simulink model "EvPowertrainController2EM_r2_23a"  (R2023a)
settings: configuration reference "VehicleFixed10ms" (kept outside this file)
model workspace (MAT data in the model file):
  CtrlVcuAccelTrqScaleFctr = [0 0.5 0.8 1 1]
  CtrlVcuBattPnlty = 10000000
  CtrlVcuBattSOCBpts = [0 20 60 80 100]
  CtrlVcuCnstrntPnltyFctr = 10000000
  CtrlVcuEMPnlty = 100
  CtrlVcuEMTrqSplitGrid = 200
  CtrlVcuMaxAccelG = 1
  CtrlVcuMaxDecelG = -1.5
  CtrlVcuPwrDeltaPnlty = 10
  CtrlVcuRegenTrqScaleFctr = [1 0.8 0.5 0.3 0]
  CtrlVcuRoadMuEst = 0.8
  CtrlVcuSftyFctr = 0.9
  CtrlVcuTracPwrErrPnlty = 6
  CtrlVcuTrqVecBrkThresh = 0.01
  CtrlVcuTrqVecIGain = 0
  CtrlVcuTrqVecMinTrq = 25
  CtrlVcuTrqVecPGain = -2000
  CtrlVcuTrqVecSteerThresh = 0.349065850399
  CtrlVcuTrqVecVelThresh = 2.5
  N_P0 = 3
undefined symbols (not defined in the file): CtrlVcuEvChrgLmtBpt, CtrlVcuEvRegenBrkCutOff, CtrlVcuEvSocBpt, eff, EnvGrvty, PlntBrkActrBoreFrnt, PlntBrkFrntBias, PlntBrkKinFricCffFrnt, PlntBrkNumPadsFrnt, PlntBrkPadMeanRadiusFrnt, PlntBrkPrsFctr, PlntBrkRearBias, PlntDiffrntl2Eff, PlntDiffrntl2Ratio, PlntDiffrntlEff, PlntDiffrntlRatio, PlntEM1EffTbl, PlntEM1Spd, PlntEM1Trq, PlntEM1TrqEff, PlntEM2EffTbl, PlntEM2Spd, PlntEM2Trq, PlntEM2TrqEff, PlntEM3EffTbl, PlntEM3Spd, PlntEM3Trq, PlntEM3TrqEff, PlntEMWhlGearEffFL, PlntEMWhlGearEffRL, PlntEMWhlGearRatioFL, PlntEMWhlGearRatioRL, PlntTransEffSpdBpt, PlntTransEffTbl, PlntTransEffTempBpt, PlntTransEffTrqBpt, PlntTransGearNumVect, PlntTransGearRatioVect, PlntVehCGHgtAxl, PlntVehDstCGFrntAxl, PlntVehDstCGRearAxl, PlntVehMass, PlntWhlLdRadius, RegenEnd, RegenStrt
libraries: simulink x28, autolibutils x4, slpidlib x2
(part 5 of 6)

== system EvPowertrainController2EM_r2_23a/Energy Management/Calculate Average EMSpd and Wheel Torque Curves for Front and Rear Axles/2EM/EMTrq2WhlTrqRear/Transmission/Diff Eta ==
  SpdIn : Inport
  TrqIn : Inport  Port=2
  Constant : Constant  Value=PlntDiffrntl2Eff
  Constant1 : Constant  SampleTime=-1
  Constant2 : Constant  Value=-1  SampleTime=-1
  Math Function1 : Math  Operator=pow  SignedPower=on  OutputSignalType=real
  Product1 : Product
  Switch2 : Switch  SaturateOnIntegerOverflow=off  InputSameDT=off
  eta : Outport  VectorParamsAs1DForOutWhenUnconnected=off
  wires:
  TrqIn/1 -> Product1/1
  Math Function1/1 -> eta/1
  Switch2/1 -> Math Function1/2
  Product1/1 -> Switch2/2
  Constant1/1 -> Switch2/1
  Constant2/1 -> Switch2/3
  Constant/1 -> Math Function1/1
  SpdIn/1 -> Product1/2

== system EvPowertrainController2EM_r2_23a/Energy Management/Calculate Average EMSpd and Wheel Torque Curves for Front and Rear Axles/2EM/EMTrq2WhlTrqRear/Transmission/Trans Eta ==
  TrqIn : Inport
  SpdIn : Inport  Port=2
  Gear : Inport  Port=3
  Abs1 : Abs  SaturateOnIntegerOverflow=off
  Constant : Constant  Value=PlntTransEffTempBpt(1)
  Constant1 : Constant  SampleTime=-1
  Constant2 : Constant  Value=-1  SampleTime=-1
  Eta 4D : Lookup_n-D  NumberOfTableDimensions=4  LookupTableObject=''  BreakpointsForDimension1=PlntTransEffTrqBpt  BreakpointsForDimension2=PlntTransEffSpdBpt  BreakpointsForDimension3=PlntTransGearNumVect  BreakpointsForDimension4=PlntTransEffTempBpt  Table=PlntTransEffTbl  ExtrapMethod=Clip  InternalRulePriority=Speed  RndMeth=Simplest
      settings: InputPortMap=u0,u1,u2,u3
  Math Function1 : Math  Operator=pow  SignedPower=on  OutputSignalType=real
  Product1 : Product
  Switch2 : Switch  SaturateOnIntegerOverflow=off  InputSameDT=off
  eta : Outport  VectorParamsAs1DForOutWhenUnconnected=off
  wires:
  Constant/1 -> Eta 4D/4
  Gear/1 -> Eta 4D/3
  SpdIn/1 -> Eta 4D/2, Product1/2
  Eta 4D/1 -> Math Function1/1
  Constant2/1 -> Switch2/3
  Constant1/1 -> Switch2/1
  Product1/1 -> Switch2/2
  Switch2/1 -> Math Function1/2
  Abs1/1 -> Eta 4D/1
  Math Function1/1 -> eta/1
  TrqIn/1 -> Abs1/1, Product1/1

== system EvPowertrainController2EM_r2_23a/Energy Management/Calculate Average EMSpd and Wheel Torque Curves for Front and Rear Axles/3EM Dual Front/EMTrq2WhlTrqFrnt/No Transmission/Gear Eta ==
  note: Pwr >= 0, v = 1
      | Pwr < 0, v= -1
  SpdIn : Inport
  TrqIn : Inport  Port=2
  Constant : Constant  Value=PlntEMWhlGearEffFL
  Constant1 : Constant  SampleTime=-1
  Constant2 : Constant  Value=-1  SampleTime=-1
  Math Function1 : Math  Operator=pow  SignedPower=on  OutputSignalType=real
  Product1 : Product
  Switch2 : Switch  SaturateOnIntegerOverflow=off  InputSameDT=off
  eta : Outport  VectorParamsAs1DForOutWhenUnconnected=off
  wires:
  TrqIn/1 -> Product1/1
  Math Function1/1 -> eta/1
  Switch2/1 -> Math Function1/2
  Product1/1 -> Switch2/2
  Constant1/1 -> Switch2/1
  Constant2/1 -> Switch2/3
  Constant/1 -> Math Function1/1
  SpdIn/1 -> Product1/2

== system EvPowertrainController2EM_r2_23a/Energy Management/Calculate Average EMSpd and Wheel Torque Curves for Front and Rear Axles/3EM Dual Front/EMTrq2WhlTrqFrnt/Transmission/Diff Eta ==
  SpdIn : Inport
  TrqIn : Inport  Port=2
  Constant : Constant  Value=PlntDiffrntlEff
  Constant1 : Constant  SampleTime=-1
  Constant2 : Constant  Value=-1  SampleTime=-1
  Math Function1 : Math  Operator=pow  SignedPower=on  OutputSignalType=real
  Product1 : Product
  Switch2 : Switch  SaturateOnIntegerOverflow=off  InputSameDT=off
  eta : Outport  VectorParamsAs1DForOutWhenUnconnected=off
  wires:
  TrqIn/1 -> Product1/1
  Math Function1/1 -> eta/1
  Switch2/1 -> Math Function1/2
  Product1/1 -> Switch2/2
  Constant1/1 -> Switch2/1
  Constant2/1 -> Switch2/3
  Constant/1 -> Math Function1/1
  SpdIn/1 -> Product1/2

== system EvPowertrainController2EM_r2_23a/Energy Management/Calculate Average EMSpd and Wheel Torque Curves for Front and Rear Axles/3EM Dual Front/EMTrq2WhlTrqFrnt/Transmission/Trans Eta ==
  TrqIn : Inport
  SpdIn : Inport  Port=2
  Gear : Inport  Port=3
  Abs1 : Abs  SaturateOnIntegerOverflow=off
  Constant : Constant  Value=PlntTransEffTempBpt(1)
  Constant1 : Constant  SampleTime=-1
  Constant2 : Constant  Value=-1  SampleTime=-1
  Eta 4D : Lookup_n-D  NumberOfTableDimensions=4  LookupTableObject=''  BreakpointsForDimension1=PlntTransEffTrqBpt  BreakpointsForDimension2=PlntTransEffSpdBpt  BreakpointsForDimension3=PlntTransGearNumVect  BreakpointsForDimension4=PlntTransEffTempBpt  Table=PlntTransEffTbl  ExtrapMethod=Clip  InternalRulePriority=Speed  RndMeth=Simplest
      settings: InputPortMap=u0,u1,u2,u3
  Math Function1 : Math  Operator=pow  SignedPower=on  OutputSignalType=real
  Product1 : Product
  Switch2 : Switch  SaturateOnIntegerOverflow=off  InputSameDT=off
  eta : Outport  VectorParamsAs1DForOutWhenUnconnected=off
  wires:
  Constant/1 -> Eta 4D/4
  Gear/1 -> Eta 4D/3
  SpdIn/1 -> Eta 4D/2, Product1/2
  Eta 4D/1 -> Math Function1/1
  Constant2/1 -> Switch2/3
  Constant1/1 -> Switch2/1
  Product1/1 -> Switch2/2
  Switch2/1 -> Math Function1/2
  Abs1/1 -> Eta 4D/1
  Math Function1/1 -> eta/1
  TrqIn/1 -> Abs1/1, Product1/1

== system EvPowertrainController2EM_r2_23a/Energy Management/Calculate Average EMSpd and Wheel Torque Curves for Front and Rear Axles/3EM Dual Front/EMTrq2WhlTrqRear/No Transmission/Diff Eta ==
  note: Pwr >= 0, v = 1
      | Pwr < 0, v= -1
  SpdIn : Inport
  TrqIn : Inport  Port=2
  Constant : Constant  Value=PlntDiffrntl2Eff
  Constant1 : Constant  SampleTime=-1
  Constant2 : Constant  Value=-1  SampleTime=-1
  Math Function1 : Math  Operator=pow  SignedPower=on  OutputSignalType=real
  Product1 : Product
  Switch2 : Switch  SaturateOnIntegerOverflow=off  InputSameDT=off
  eta : Outport  VectorParamsAs1DForOutWhenUnconnected=off
  wires:
  TrqIn/1 -> Product1/1
  Math Function1/1 -> eta/1
  Switch2/1 -> Math Function1/2
  Product1/1 -> Switch2/2
  Constant1/1 -> Switch2/1
  Constant2/1 -> Switch2/3
  Constant/1 -> Math Function1/1
  SpdIn/1 -> Product1/2

== system EvPowertrainController2EM_r2_23a/Energy Management/Calculate Average EMSpd and Wheel Torque Curves for Front and Rear Axles/3EM Dual Front/EMTrq2WhlTrqRear/Transmission/Diff Eta ==
  SpdIn : Inport
  TrqIn : Inport  Port=2
  Constant : Constant  Value=PlntDiffrntl2Eff
  Constant1 : Constant  SampleTime=-1
  Constant2 : Constant  Value=-1  SampleTime=-1
  Math Function1 : Math  Operator=pow  SignedPower=on  OutputSignalType=real
  Product1 : Product
  Switch2 : Switch  SaturateOnIntegerOverflow=off  InputSameDT=off
  eta : Outport  VectorParamsAs1DForOutWhenUnconnected=off
  wires:
  SpdIn/1 -> Product1/2
  Constant/1 -> Math Function1/1
  Constant2/1 -> Switch2/3
  Constant1/1 -> Switch2/1
  Product1/1 -> Switch2/2
  Switch2/1 -> Math Function1/2
  Math Function1/1 -> eta/1
  TrqIn/1 -> Product1/1

== system EvPowertrainController2EM_r2_23a/Energy Management/Calculate Average EMSpd and Wheel Torque Curves for Front and Rear Axles/3EM Dual Front/EMTrq2WhlTrqRear/Transmission/Trans Eta ==
  TrqIn : Inport
  SpdIn : Inport  Port=2
  Gear : Inport  Port=3
  Abs1 : Abs  SaturateOnIntegerOverflow=off
  Constant : Constant  Value=PlntTransEffTempBpt(1)
  Constant1 : Constant  SampleTime=-1
  Constant2 : Constant  Value=-1  SampleTime=-1
  Eta 4D : Lookup_n-D  NumberOfTableDimensions=4  LookupTableObject=''  BreakpointsForDimension1=PlntTransEffTrqBpt  BreakpointsForDimension2=PlntTransEffSpdBpt  BreakpointsForDimension3=PlntTransGearNumVect  BreakpointsForDimension4=PlntTransEffTempBpt  Table=PlntTransEffTbl  ExtrapMethod=Clip  InternalRulePriority=Speed  RndMeth=Simplest
      settings: InputPortMap=u0,u1,u2,u3
  Math Function1 : Math  Operator=pow  SignedPower=on  OutputSignalType=real
  Product1 : Product
  Switch2 : Switch  SaturateOnIntegerOverflow=off  InputSameDT=off
  eta : Outport  VectorParamsAs1DForOutWhenUnconnected=off
  wires:
  TrqIn/1 -> Product1/1, Abs1/1
  Math Function1/1 -> eta/1
  Abs1/1 -> Eta 4D/1
  Switch2/1 -> Math Function1/2
  Product1/1 -> Switch2/2
  Constant1/1 -> Switch2/1
  Constant2/1 -> Switch2/3
  Eta 4D/1 -> Math Function1/1
  SpdIn/1 -> Product1/2, Eta 4D/2
  Gear/1 -> Eta 4D/3
  Constant/1 -> Eta 4D/4

== system EvPowertrainController2EM_r2_23a/Energy Management/Calculate Average EMSpd and Wheel Torque Curves for Front and Rear Axles/3EM Dual Rear/EMTrq2WhlTrqFrnt/No Transmission/Diff Eta ==
  note: Pwr >= 0, v = 1
      | Pwr < 0, v= -1
  SpdIn : Inport
  TrqIn : Inport  Port=2
  Constant : Constant  Value=PlntDiffrntlEff
  Constant1 : Constant  SampleTime=-1
  Constant2 : Constant  Value=-1  SampleTime=-1
  Math Function1 : Math  Operator=pow  SignedPower=on  OutputSignalType=real
  Product1 : Product
  Switch2 : Switch  SaturateOnIntegerOverflow=off  InputSameDT=off
  eta : Outport  VectorParamsAs1DForOutWhenUnconnected=off
  wires:
  SpdIn/1 -> Product1/2
  Constant/1 -> Math Function1/1
  Constant2/1 -> Switch2/3
  Constant1/1 -> Switch2/1
  Product1/1 -> Switch2/2
  Switch2/1 -> Math Function1/2
  Math Function1/1 -> eta/1
  TrqIn/1 -> Product1/1

== system EvPowertrainController2EM_r2_23a/Energy Management/Calculate Average EMSpd and Wheel Torque Curves for Front and Rear Axles/3EM Dual Rear/EMTrq2WhlTrqFrnt/Transmission/Diff Eta ==
  SpdIn : Inport
  TrqIn : Inport  Port=2
  Constant : Constant  Value=PlntDiffrntlEff
  Constant1 : Constant  SampleTime=-1
  Constant2 : Constant  Value=-1  SampleTime=-1
  Math Function1 : Math  Operator=pow  SignedPower=on  OutputSignalType=real
  Product1 : Product
  Switch2 : Switch  SaturateOnIntegerOverflow=off  InputSameDT=off
  eta : Outport  VectorParamsAs1DForOutWhenUnconnected=off
  wires:
  SpdIn/1 -> Product1/2
  Constant/1 -> Math Function1/1
  Constant2/1 -> Switch2/3
  Constant1/1 -> Switch2/1
  Product1/1 -> Switch2/2
  Switch2/1 -> Math Function1/2
  Math Function1/1 -> eta/1
  TrqIn/1 -> Product1/1

== system EvPowertrainController2EM_r2_23a/Energy Management/Calculate Average EMSpd and Wheel Torque Curves for Front and Rear Axles/3EM Dual Rear/EMTrq2WhlTrqFrnt/Transmission/Trans Eta ==
  TrqIn : Inport
  SpdIn : Inport  Port=2
  Gear : Inport  Port=3
  Abs1 : Abs  SaturateOnIntegerOverflow=off
  Constant : Constant  Value=PlntTransEffTempBpt(1)
  Constant1 : Constant  SampleTime=-1
  Constant2 : Constant  Value=-1  SampleTime=-1
  Eta 4D : Lookup_n-D  NumberOfTableDimensions=4  LookupTableObject=''  BreakpointsForDimension1=PlntTransEffTrqBpt  BreakpointsForDimension2=PlntTransEffSpdBpt  BreakpointsForDimension3=PlntTransGearNumVect  BreakpointsForDimension4=PlntTransEffTempBpt  Table=PlntTransEffTbl  ExtrapMethod=Clip  InternalRulePriority=Speed  RndMeth=Simplest
      settings: InputPortMap=u0,u1,u2,u3
  Math Function1 : Math  Operator=pow  SignedPower=on  OutputSignalType=real
  Product1 : Product
  Switch2 : Switch  SaturateOnIntegerOverflow=off  InputSameDT=off
  eta : Outport  VectorParamsAs1DForOutWhenUnconnected=off
  wires:
  TrqIn/1 -> Product1/1, Abs1/1
  Math Function1/1 -> eta/1
  Abs1/1 -> Eta 4D/1
  Switch2/1 -> Math Function1/2
  Product1/1 -> Switch2/2
  Constant1/1 -> Switch2/1
  Constant2/1 -> Switch2/3
  Eta 4D/1 -> Math Function1/1
  SpdIn/1 -> Product1/2, Eta 4D/2
  Gear/1 -> Eta 4D/3
  Constant/1 -> Eta 4D/4

== system EvPowertrainController2EM_r2_23a/Energy Management/Calculate Average EMSpd and Wheel Torque Curves for Front and Rear Axles/3EM Dual Rear/EMTrq2WhlTrqRear/No Transmission/Gear Eta ==
  note: Pwr >= 0, v = 1
      | Pwr < 0, v= -1
  SpdIn : Inport
  TrqIn : Inport  Port=2
  Constant : Constant  Value=PlntEMWhlGearEffRL
  Constant1 : Constant  SampleTime=-1
  Constant2 : Constant  Value=-1  SampleTime=-1
  Math Function1 : Math  Operator=pow  SignedPower=on  OutputSignalType=real
  Product1 : Product
  Switch2 : Switch  SaturateOnIntegerOverflow=off  InputSameDT=off
  eta : Outport  VectorParamsAs1DForOutWhenUnconnected=off
  wires:
  SpdIn/1 -> Product1/2
  Constant/1 -> Math Function1/1
  Constant2/1 -> Switch2/3
  Constant1/1 -> Switch2/1
  Product1/1 -> Switch2/2
  Switch2/1 -> Math Function1/2
  Math Function1/1 -> eta/1
  TrqIn/1 -> Product1/1

== system EvPowertrainController2EM_r2_23a/Energy Management/Calculate Average EMSpd and Wheel Torque Curves for Front and Rear Axles/3EM Dual Rear/EMTrq2WhlTrqRear/Transmission/Diff Eta ==
  SpdIn : Inport
  TrqIn : Inport  Port=2
  Constant : Constant  Value=PlntDiffrntl2Eff
  Constant1 : Constant  SampleTime=-1
  Constant2 : Constant  Value=-1  SampleTime=-1
  Math Function1 : Math  Operator=pow  SignedPower=on  OutputSignalType=real
  Product1 : Product
  Switch2 : Switch  SaturateOnIntegerOverflow=off  InputSameDT=off
  eta : Outport  VectorParamsAs1DForOutWhenUnconnected=off
  wires:
  TrqIn/1 -> Product1/1
  Math Function1/1 -> eta/1
  Switch2/1 -> Math Function1/2
  Product1/1 -> Switch2/2
  Constant1/1 -> Switch2/1
  Constant2/1 -> Switch2/3
  Constant/1 -> Math Function1/1
  SpdIn/1 -> Product1/2

== system EvPowertrainController2EM_r2_23a/Energy Management/Calculate Average EMSpd and Wheel Torque Curves for Front and Rear Axles/3EM Dual Rear/EMTrq2WhlTrqRear/Transmission/Trans Eta ==
  TrqIn : Inport
  SpdIn : Inport  Port=2
  Gear : Inport  Port=3
  Abs1 : Abs  SaturateOnIntegerOverflow=off
  Constant : Constant  Value=PlntTransEffTempBpt(1)
  Constant1 : Constant  SampleTime=-1
  Constant2 : Constant  Value=-1  SampleTime=-1
  Eta 4D : Lookup_n-D  NumberOfTableDimensions=4  LookupTableObject=''  BreakpointsForDimension1=PlntTransEffTrqBpt  BreakpointsForDimension2=PlntTransEffSpdBpt  BreakpointsForDimension3=PlntTransGearNumVect  BreakpointsForDimension4=PlntTransEffTempBpt  Table=PlntTransEffTbl  ExtrapMethod=Clip  InternalRulePriority=Speed  RndMeth=Simplest
      settings: InputPortMap=u0,u1,u2,u3
  Math Function1 : Math  Operator=pow  SignedPower=on  OutputSignalType=real
  Product1 : Product
  Switch2 : Switch  SaturateOnIntegerOverflow=off  InputSameDT=off
  eta : Outport  VectorParamsAs1DForOutWhenUnconnected=off
  wires:
  Constant/1 -> Eta 4D/4
  Gear/1 -> Eta 4D/3
  SpdIn/1 -> Eta 4D/2, Product1/2
  Eta 4D/1 -> Math Function1/1
  Constant2/1 -> Switch2/3
  Constant1/1 -> Switch2/1
  Product1/1 -> Switch2/2
  Switch2/1 -> Math Function1/2
  Abs1/1 -> Eta 4D/1
  Math Function1/1 -> eta/1
  TrqIn/1 -> Abs1/1, Product1/1

== system EvPowertrainController2EM_r2_23a/Energy Management/Calculate Average EMSpd and Wheel Torque Curves for Front and Rear Axles/4EM/EMTrq2WhlTrqFrnt/No Transmission/Gear Eta ==
  note: Pwr >= 0, v = 1
      | Pwr < 0, v= -1
  SpdIn : Inport
  TrqIn : Inport  Port=2
  Constant : Constant  Value=PlntEMWhlGearEffFL
  Constant1 : Constant  SampleTime=-1
  Constant2 : Constant  Value=-1  SampleTime=-1
  Math Function1 : Math  Operator=pow  SignedPower=on  OutputSignalType=real
  Product1 : Product
  Switch2 : Switch  SaturateOnIntegerOverflow=off  InputSameDT=off
  eta : Outport  VectorParamsAs1DForOutWhenUnconnected=off
  wires:
  TrqIn/1 -> Product1/1
  Math Function1/1 -> eta/1
  Switch2/1 -> Math Function1/2
  Product1/1 -> Switch2/2
  Constant1/1 -> Switch2/1
  Constant2/1 -> Switch2/3
  Constant/1 -> Math Function1/1
  SpdIn/1 -> Product1/2

== system EvPowertrainController2EM_r2_23a/Energy Management/Calculate Average EMSpd and Wheel Torque Curves for Front and Rear Axles/4EM/EMTrq2WhlTrqFrnt/Transmission/Diff Eta ==
  SpdIn : Inport
  TrqIn : Inport  Port=2
  Constant : Constant  Value=PlntDiffrntlEff
  Constant1 : Constant  SampleTime=-1
  Constant2 : Constant  Value=-1  SampleTime=-1
  Math Function1 : Math  Operator=pow  SignedPower=on  OutputSignalType=real
  Product1 : Product
  Switch2 : Switch  SaturateOnIntegerOverflow=off  InputSameDT=off
  eta : Outport  VectorParamsAs1DForOutWhenUnconnected=off
  wires:
  TrqIn/1 -> Product1/1
  Math Function1/1 -> eta/1
  Switch2/1 -> Math Function1/2
  Product1/1 -> Switch2/2
  Constant1/1 -> Switch2/1
  Constant2/1 -> Switch2/3
  Constant/1 -> Math Function1/1
  SpdIn/1 -> Product1/2

== system EvPowertrainController2EM_r2_23a/Energy Management/Calculate Average EMSpd and Wheel Torque Curves for Front and Rear Axles/4EM/EMTrq2WhlTrqFrnt/Transmission/Trans Eta ==
  TrqIn : Inport
  SpdIn : Inport  Port=2
  Gear : Inport  Port=3
  Abs1 : Abs  SaturateOnIntegerOverflow=off
  Constant : Constant  Value=PlntTransEffTempBpt(1)
  Constant1 : Constant  SampleTime=-1
  Constant2 : Constant  Value=-1  SampleTime=-1
  Eta 4D : Lookup_n-D  NumberOfTableDimensions=4  LookupTableObject=''  BreakpointsForDimension1=PlntTransEffTrqBpt  BreakpointsForDimension2=PlntTransEffSpdBpt  BreakpointsForDimension3=PlntTransGearNumVect  BreakpointsForDimension4=PlntTransEffTempBpt  Table=PlntTransEffTbl  ExtrapMethod=Clip  InternalRulePriority=Speed  RndMeth=Simplest
      settings: InputPortMap=u0,u1,u2,u3
  Math Function1 : Math  Operator=pow  SignedPower=on  OutputSignalType=real
  Product1 : Product
  Switch2 : Switch  SaturateOnIntegerOverflow=off  InputSameDT=off
  eta : Outport  VectorParamsAs1DForOutWhenUnconnected=off
  wires:
  Constant/1 -> Eta 4D/4
  Gear/1 -> Eta 4D/3
  SpdIn/1 -> Eta 4D/2, Product1/2
  Eta 4D/1 -> Math Function1/1
  Constant2/1 -> Switch2/3
  Constant1/1 -> Switch2/1
  Product1/1 -> Switch2/2
  Switch2/1 -> Math Function1/2
  Abs1/1 -> Eta 4D/1
  Math Function1/1 -> eta/1
  TrqIn/1 -> Abs1/1, Product1/1

== system EvPowertrainController2EM_r2_23a/Energy Management/Calculate Average EMSpd and Wheel Torque Curves for Front and Rear Axles/4EM/EMTrq2WhlTrqRear/No Transmission/Gear Eta ==
  note: Pwr >= 0, v = 1
      | Pwr < 0, v= -1
  SpdIn : Inport
  TrqIn : Inport  Port=2
  Constant : Constant  Value=PlntEMWhlGearEffRL
  Constant1 : Constant  SampleTime=-1
  Constant2 : Constant  Value=-1  SampleTime=-1
  Math Function1 : Math  Operator=pow  SignedPower=on  OutputSignalType=real
  Product1 : Product
  Switch2 : Switch  SaturateOnIntegerOverflow=off  InputSameDT=off
  eta : Outport  VectorParamsAs1DForOutWhenUnconnected=off
  wires:
  TrqIn/1 -> Product1/1
  Math Function1/1 -> eta/1
  Switch2/1 -> Math Function1/2
  Product1/1 -> Switch2/2
  Constant1/1 -> Switch2/1
  Constant2/1 -> Switch2/3
  Constant/1 -> Math Function1/1
  SpdIn/1 -> Product1/2

== system EvPowertrainController2EM_r2_23a/Energy Management/Calculate Average EMSpd and Wheel Torque Curves for Front and Rear Axles/4EM/EMTrq2WhlTrqRear/Transmission/Diff Eta ==
  SpdIn : Inport
  TrqIn : Inport  Port=2
  Constant : Constant  Value=PlntDiffrntl2Eff
  Constant1 : Constant  SampleTime=-1
  Constant2 : Constant  Value=-1  SampleTime=-1
  Math Function1 : Math  Operator=pow  SignedPower=on  OutputSignalType=real
  Product1 : Product
  Switch2 : Switch  SaturateOnIntegerOverflow=off  InputSameDT=off
  eta : Outport  VectorParamsAs1DForOutWhenUnconnected=off
  wires:
  SpdIn/1 -> Product1/2
  Constant/1 -> Math Function1/1
  Constant2/1 -> Switch2/3
  Constant1/1 -> Switch2/1
  Product1/1 -> Switch2/2
  Switch2/1 -> Math Function1/2
  Math Function1/1 -> eta/1
  TrqIn/1 -> Product1/1

== system EvPowertrainController2EM_r2_23a/Energy Management/Calculate Average EMSpd and Wheel Torque Curves for Front and Rear Axles/4EM/EMTrq2WhlTrqRear/Transmission/Trans Eta ==
  TrqIn : Inport
  SpdIn : Inport  Port=2
  Gear : Inport  Port=3
  Abs1 : Abs  SaturateOnIntegerOverflow=off
  Constant : Constant  Value=PlntTransEffTempBpt(1)
  Constant1 : Constant  SampleTime=-1
  Constant2 : Constant  Value=-1  SampleTime=-1
  Eta 4D : Lookup_n-D  NumberOfTableDimensions=4  LookupTableObject=''  BreakpointsForDimension1=PlntTransEffTrqBpt  BreakpointsForDimension2=PlntTransEffSpdBpt  BreakpointsForDimension3=PlntTransGearNumVect  BreakpointsForDimension4=PlntTransEffTempBpt  Table=PlntTransEffTbl  ExtrapMethod=Clip  InternalRulePriority=Speed  RndMeth=Simplest
      settings: InputPortMap=u0,u1,u2,u3
  Math Function1 : Math  Operator=pow  SignedPower=on  OutputSignalType=real
  Product1 : Product
  Switch2 : Switch  SaturateOnIntegerOverflow=off  InputSameDT=off
  eta : Outport  VectorParamsAs1DForOutWhenUnconnected=off
  wires:
  TrqIn/1 -> Product1/1, Abs1/1
  Math Function1/1 -> eta/1
  Abs1/1 -> Eta 4D/1
  Switch2/1 -> Math Function1/2
  Product1/1 -> Switch2/2
  Constant1/1 -> Switch2/1
  Constant2/1 -> Switch2/3
  Eta 4D/1 -> Math Function1/1
  SpdIn/1 -> Product1/2, Eta 4D/2
  Gear/1 -> Eta 4D/3
  Constant/1 -> Eta 4D/4

== system EvPowertrainController2EM_r2_23a/Energy Management/Powertrain Constraints /Battery Constraint/Electrical Current/DC-DC Eta/DC-DC Eta ==
  In : Inport
  DCDC Constant Eff : Gain  Gain=1+(100-eff)/100
  Out : Outport  VectorParamsAs1DForOutWhenUnconnected=off
  wires:
  DCDC Constant Eff/1 -> Out/1
  In/1 -> DCDC Constant Eff/1

== system EvPowertrainController2EM_r2_23a/Energy Management/Powertrain Constraints /Battery Constraint/Electrical Current/DC-DC Eta/No DC-DC ==
  In : Inport
  Out : Outport  VectorParamsAs1DForOutWhenUnconnected=off
  wires:
  In/1 -> Out/1

== system EvPowertrainController2EM_r2_23a/Energy Management/Powertrain Constraints /EM Constraint Front/Tabular Power Loss Data/2EM or 3EM Dual Rear/WhlTrq2EMTrq ==
  EMSpd : Inport
  WhlTrqCmd : Inport  Port=2
  Diff Eta : Subsystem
  Divide2 : Product  Inputs=/*
  Gain3 : Gain  Gain=1/PlntDiffrntlRatio
  Unit Delay : UnitDelay  SampleTime=-1  HasFrameUpgradeWarning=on
  EMTrq : Outport  VectorParamsAs1DForOutWhenUnconnected=off
  wires:
  Unit Delay/1 -> Diff Eta/2(TrqIn)
  Diff Eta/1(eta) -> Divide2/1
  WhlTrqCmd/1 -> Gain3/1
  EMSpd/1 -> Diff Eta/1(SpdIn)
  Divide2/1 -> EMTrq/1, Unit Delay/1
  Gain3/1 -> Divide2/2

== system EvPowertrainController2EM_r2_23a/Energy Management/Powertrain Constraints /EM Constraint Front/Tabular Power Loss Data/3EM Dual Front or 4EM/WhlTrq2EMTrq ==
  EMSpd : Inport
  WhlTrqCmd : Inport  Port=2
  Divide2 : Product  Inputs=/*
  Dual EMs : Gain  Gain=1/2
  Gain3 : Gain  Gain=1/PlntEMWhlGearRatioFL
  Gear Eta : Subsystem
  Unit Delay : UnitDelay  SampleTime=-1  HasFrameUpgradeWarning=on
  EMTrq : Outport  VectorParamsAs1DForOutWhenUnconnected=off
  wires:
  Dual EMs/1 -> Gain3/1
  Gain3/1 -> Divide2/2
  Divide2/1 -> Unit Delay/1, EMTrq/1
  EMSpd/1 -> Gear Eta/1(SpdIn)
  WhlTrqCmd/1 -> Dual EMs/1
  Gear Eta/1(eta) -> Divide2/1
  Unit Delay/1 -> Gear Eta/2(TrqIn)

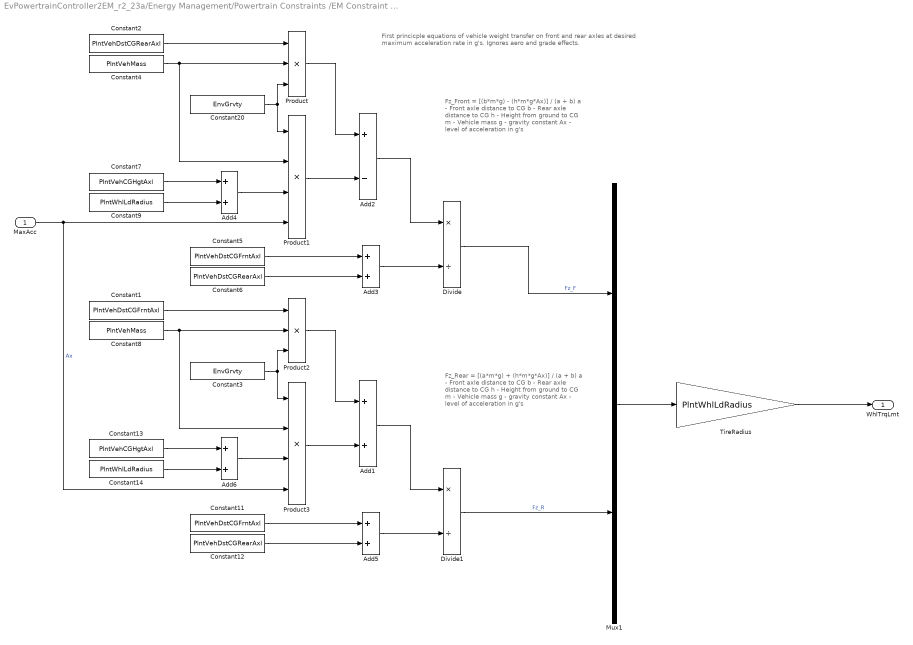
== system EvPowertrainController2EM_r2_23a/Energy Management/Powertrain Constraints /EM Constraint Front/Wheel Torque Saturation for Max g Rates1/Wheel Torque Limit at Max g Rates/Wheel Torque at Max Acceleration Rate ==
  note: Fz_Rear = [(a*m*g) + (h*m*g*Ax)] / (a + b)
      |
      | a - Front axle distance to CG
      | b - Rear axle distance to CG
      | h - Height from ground to CG
      | m - Vehicle mass
      | g - gravity constant
      | Ax - level of acceleration in g's
  note: Fz_Front = [(b*m*g) - (h*m*g*Ax)] / (a + b)
      |
      | a - Front axle distance to CG
      | b - Rear axle distance to CG
      | h - Height from ground to CG
      | m - Vehicle mass
      | g - gravity constant
      | Ax - level of acceleration in g's
  note: First princicple equations of vehicle weight transfer on front
      | and rear axles at desired maximum acceleration rate in g's.
      | Ignores aero and grade effects.
  MaxAcc : Inport
  Add{1,3..6} (5 alike) : Sum
  Add2 : Sum  Inputs=+-
  Constant1 : Constant  Value=PlntVehDstCGFrntAxl  SampleTime=-1
  Constant11 : Constant  Value=PlntVehDstCGFrntAxl  SampleTime=-1
  Constant12 : Constant  Value=PlntVehDstCGRearAxl  SampleTime=-1
  Constant13 : Constant  Value=PlntVehCGHgtAxl  SampleTime=-1
  Constant14 : Constant  Value=PlntWhlLdRadius  SampleTime=-1
  Constant2 : Constant  Value=PlntVehDstCGRearAxl  SampleTime=-1
  Constant20 : Constant  Value=EnvGrvty  SampleTime=-1
  Constant3 : Constant  Value=EnvGrvty  SampleTime=-1
  Constant4 : Constant  Value=PlntVehMass  SampleTime=-1
  Constant5 : Constant  Value=PlntVehDstCGFrntAxl  SampleTime=-1
  Constant6 : Constant  Value=PlntVehDstCGRearAxl  SampleTime=-1
  Constant7 : Constant  Value=PlntVehCGHgtAxl  SampleTime=-1
  Constant8 : Constant  Value=PlntVehMass  SampleTime=-1
  Constant9 : Constant  Value=PlntWhlLdRadius  SampleTime=-1
  Divide : Product  Inputs=*/
  Divide1 : Product  Inputs=*/
  Mux1 : Mux  Inputs=2
  Product : Product  Inputs=3
  Product1 : Product  Inputs=4
  Product2 : Product  Inputs=3
  Product3 : Product  Inputs=4
  TireRadius : Gain  Gain=PlntWhlLdRadius
  WhlTrqLmt : Outport  VectorParamsAs1DForOutWhenUnconnected=off
  wires:
  Divide1/1 -> Mux1/2  "Fz_R"
  Product3/1 -> Add1/2
  Product2/1 -> Add1/1
  Constant11/1 -> Add5/1
  Constant8/1 -> Product3/2, Product2/2
  Add5/1 -> Divide1/2
  Add6/1 -> Product3/3
  Constant12/1 -> Add5/2
  Constant1/1 -> Product2/1
  Constant13/1 -> Add6/1
  Constant14/1 -> Add6/2
  Add1/1 -> Divide1/1
  Constant3/1 -> Product3/1, Product2/3
  Constant20/1 -> Product/3, Product1/1
  TireRadius/1 -> WhlTrqLmt/1
  Add2/1 -> Divide/1
  Constant9/1 -> Add4/2
  Constant7/1 -> Add4/1
  Constant2/1 -> Product/1
  Constant6/1 -> Add3/2
  Mux1/1 -> TireRadius/1
  Divide/1 -> Mux1/1  "Fz_F"
  Add4/1 -> Product1/3
  Add3/1 -> Divide/2
  MaxAcc/1 -> Product1/4, Product3/4  "Ax"
  Constant4/1 -> Product/2, Product1/2
  Constant5/1 -> Add3/1
  Product/1 -> Add2/1
  Product1/1 -> Add2/2

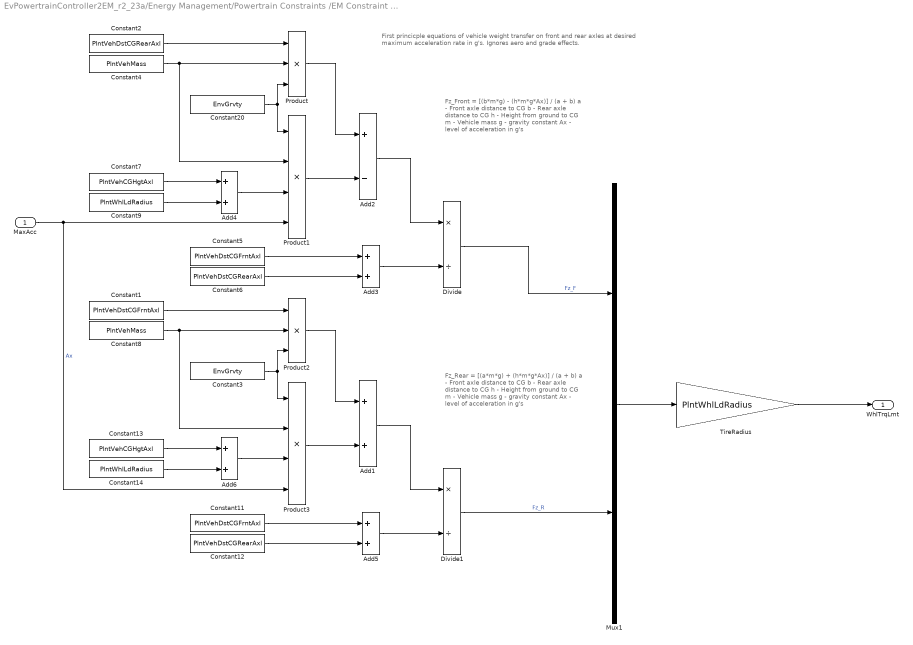
== system EvPowertrainController2EM_r2_23a/Energy Management/Powertrain Constraints /EM Constraint Front/Wheel Torque Saturation for Max g Rates1/Wheel Torque Limit at Max g Rates/Wheel Torque at Max Deceleration Rate ==
  note: First princicple equations of vehicle weight transfer on front
      | and rear axles at desired maximum acceleration rate in g's.
      | Ignores aero and grade effects.
  note: Fz_Front = [(b*m*g) - (h*m*g*Ax)] / (a + b)
      |
      | a - Front axle distance to CG
      | b - Rear axle distance to CG
      | h - Height from ground to CG
      | m - Vehicle mass
      | g - gravity constant
      | Ax - level of acceleration in g's
  note: Fz_Rear = [(a*m*g) + (h*m*g*Ax)] / (a + b)
      |
      | a - Front axle distance to CG
      | b - Rear axle distance to CG
      | h - Height from ground to CG
      | m - Vehicle mass
      | g - gravity constant
      | Ax - level of acceleration in g's
  MaxAcc : Inport
  Add{1,3..6} (5 alike) : Sum
  Add2 : Sum  Inputs=+-
  Constant1 : Constant  Value=PlntVehDstCGFrntAxl  SampleTime=-1
  Constant11 : Constant  Value=PlntVehDstCGFrntAxl  SampleTime=-1
  Constant12 : Constant  Value=PlntVehDstCGRearAxl  SampleTime=-1
  Constant13 : Constant  Value=PlntVehCGHgtAxl  SampleTime=-1
  Constant14 : Constant  Value=PlntWhlLdRadius  SampleTime=-1
  Constant2 : Constant  Value=PlntVehDstCGRearAxl  SampleTime=-1
  Constant20 : Constant  Value=EnvGrvty  SampleTime=-1
  Constant3 : Constant  Value=EnvGrvty  SampleTime=-1
  Constant4 : Constant  Value=PlntVehMass  SampleTime=-1
  Constant5 : Constant  Value=PlntVehDstCGFrntAxl  SampleTime=-1
  Constant6 : Constant  Value=PlntVehDstCGRearAxl  SampleTime=-1
  Constant7 : Constant  Value=PlntVehCGHgtAxl  SampleTime=-1
  Constant8 : Constant  Value=PlntVehMass  SampleTime=-1
  Constant9 : Constant  Value=PlntWhlLdRadius  SampleTime=-1
  Divide : Product  Inputs=*/
  Divide1 : Product  Inputs=*/
  Mux1 : Mux  Inputs=2
  Product : Product  Inputs=3
  Product1 : Product  Inputs=4
  Product2 : Product  Inputs=3
  Product3 : Product  Inputs=4
  TireRadius : Gain  Gain=PlntWhlLdRadius
  WhlTrqLmt : Outport  VectorParamsAs1DForOutWhenUnconnected=off
  wires:
  Product1/1 -> Add2/2
  Product/1 -> Add2/1
  Constant5/1 -> Add3/1
  Constant4/1 -> Product1/2, Product/2
  MaxAcc/1 -> Product3/4, Product1/4  "Ax"
  Add3/1 -> Divide/2
  Add4/1 -> Product1/3
  Divide/1 -> Mux1/1  "Fz_F"
  Mux1/1 -> TireRadius/1
  Constant6/1 -> Add3/2
  Constant2/1 -> Product/1
  Constant7/1 -> Add4/1
  Constant9/1 -> Add4/2
  Add2/1 -> Divide/1
  TireRadius/1 -> WhlTrqLmt/1
  Constant20/1 -> Product1/1, Product/3
  Constant3/1 -> Product2/3, Product3/1
  Add1/1 -> Divide1/1
  Constant14/1 -> Add6/2
  Constant13/1 -> Add6/1
  Constant1/1 -> Product2/1
  Constant12/1 -> Add5/2
  Add6/1 -> Product3/3
  Add5/1 -> Divide1/2
  Constant8/1 -> Product2/2, Product3/2
  Constant11/1 -> Add5/1
  Product2/1 -> Add1/1
  Product3/1 -> Add1/2
  Divide1/1 -> Mux1/2  "Fz_R"

== system EvPowertrainController2EM_r2_23a/Energy Management/Powertrain Constraints /EM Constraint Rear/Tabular Power Loss Data/2EM/WhlTrq2EMTrq ==
  EMSpd : Inport
  WhlTrqCmd : Inport  Port=2
  Diff Eta : Subsystem
  Divide2 : Product  Inputs=/*
  Gain3 : Gain  Gain=1/PlntDiffrntl2Ratio
  Unit Delay : UnitDelay  SampleTime=-1  HasFrameUpgradeWarning=on
  EMTrq : Outport  VectorParamsAs1DForOutWhenUnconnected=off
  wires:
  Unit Delay/1 -> Diff Eta/2(TrqIn)
  Diff Eta/1(eta) -> Divide2/1
  WhlTrqCmd/1 -> Gain3/1
  EMSpd/1 -> Diff Eta/1(SpdIn)
  Divide2/1 -> EMTrq/1, Unit Delay/1
  Gain3/1 -> Divide2/2

== system EvPowertrainController2EM_r2_23a/Energy Management/Powertrain Constraints /EM Constraint Rear/Tabular Power Loss Data/3EM Dual Front/WhlTrq2EMTrq ==
  EMSpd : Inport
  WhlTrqCmd : Inport  Port=2
  Diff Eta : Subsystem
  Divide2 : Product  Inputs=/*
  Gain3 : Gain  Gain=1/PlntDiffrntl2Ratio
  Unit Delay : UnitDelay  SampleTime=-1  HasFrameUpgradeWarning=on
  EMTrq : Outport  VectorParamsAs1DForOutWhenUnconnected=off
  wires:
  Gain3/1 -> Divide2/2
  Divide2/1 -> Unit Delay/1, EMTrq/1
  EMSpd/1 -> Diff Eta/1(SpdIn)
  WhlTrqCmd/1 -> Gain3/1
  Diff Eta/1(eta) -> Divide2/1
  Unit Delay/1 -> Diff Eta/2(TrqIn)

== system EvPowertrainController2EM_r2_23a/Energy Management/Powertrain Constraints /EM Constraint Rear/Tabular Power Loss Data/3EM Dual Rear or 4EM/WhlTrq2EMTrq ==
  EMSpd : Inport
  WhlTrqCmd : Inport  Port=2
  Divide2 : Product  Inputs=/*
  Dual EMs : Gain  Gain=1/2
  Gain3 : Gain  Gain=1/PlntEMWhlGearRatioRL
  Gear Eta : Subsystem
  Unit Delay : UnitDelay  SampleTime=-1  HasFrameUpgradeWarning=on
  EMTrq : Outport  VectorParamsAs1DForOutWhenUnconnected=off
  wires:
  Dual EMs/1 -> Gain3/1
  Gain3/1 -> Divide2/2
  Divide2/1 -> Unit Delay/1, EMTrq/1
  EMSpd/1 -> Gear Eta/1(SpdIn)
  WhlTrqCmd/1 -> Dual EMs/1
  Gear Eta/1(eta) -> Divide2/1
  Unit Delay/1 -> Gear Eta/2(TrqIn)

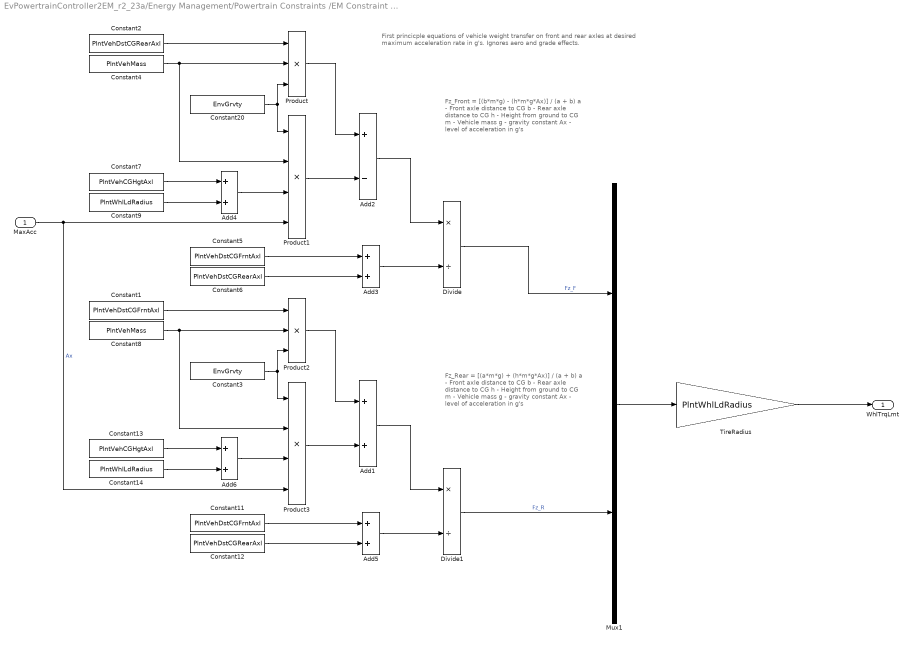
== system EvPowertrainController2EM_r2_23a/Energy Management/Powertrain Constraints /EM Constraint Rear/Wheel Torque Saturation for Max g Rates/Wheel Torque Limit at Max g Rates/Wheel Torque at Max Acceleration Rate ==
  note: Fz_Rear = [(a*m*g) + (h*m*g*Ax)] / (a + b)
      |
      | a - Front axle distance to CG
      | b - Rear axle distance to CG
      | h - Height from ground to CG
      | m - Vehicle mass
      | g - gravity constant
      | Ax - level of acceleration in g's
  note: Fz_Front = [(b*m*g) - (h*m*g*Ax)] / (a + b)
      |
      | a - Front axle distance to CG
      | b - Rear axle distance to CG
      | h - Height from ground to CG
      | m - Vehicle mass
      | g - gravity constant
      | Ax - level of acceleration in g's
  note: First princicple equations of vehicle weight transfer on front
      | and rear axles at desired maximum acceleration rate in g's.
      | Ignores aero and grade effects.
  MaxAcc : Inport
  Add{1,3..6} (5 alike) : Sum
  Add2 : Sum  Inputs=+-
  Constant1 : Constant  Value=PlntVehDstCGFrntAxl  SampleTime=-1
  Constant11 : Constant  Value=PlntVehDstCGFrntAxl  SampleTime=-1
  Constant12 : Constant  Value=PlntVehDstCGRearAxl  SampleTime=-1
  Constant13 : Constant  Value=PlntVehCGHgtAxl  SampleTime=-1
  Constant14 : Constant  Value=PlntWhlLdRadius  SampleTime=-1
  Constant2 : Constant  Value=PlntVehDstCGRearAxl  SampleTime=-1
  Constant20 : Constant  Value=EnvGrvty  SampleTime=-1
  Constant3 : Constant  Value=EnvGrvty  SampleTime=-1
  Constant4 : Constant  Value=PlntVehMass  SampleTime=-1
  Constant5 : Constant  Value=PlntVehDstCGFrntAxl  SampleTime=-1
  Constant6 : Constant  Value=PlntVehDstCGRearAxl  SampleTime=-1
  Constant7 : Constant  Value=PlntVehCGHgtAxl  SampleTime=-1
  Constant8 : Constant  Value=PlntVehMass  SampleTime=-1
  Constant9 : Constant  Value=PlntWhlLdRadius  SampleTime=-1
  Divide : Product  Inputs=*/
  Divide1 : Product  Inputs=*/
  Mux1 : Mux  Inputs=2
  Product : Product  Inputs=3
  Product1 : Product  Inputs=4
  Product2 : Product  Inputs=3
  Product3 : Product  Inputs=4
  TireRadius : Gain  Gain=PlntWhlLdRadius
  WhlTrqLmt : Outport  VectorParamsAs1DForOutWhenUnconnected=off
  wires:
  Divide1/1 -> Mux1/2  "Fz_R"
  Product3/1 -> Add1/2
  Product2/1 -> Add1/1
  Constant11/1 -> Add5/1
  Constant8/1 -> Product3/2, Product2/2
  Add5/1 -> Divide1/2
  Add6/1 -> Product3/3
  Constant12/1 -> Add5/2
  Constant1/1 -> Product2/1
  Constant13/1 -> Add6/1
  Constant14/1 -> Add6/2
  Add1/1 -> Divide1/1
  Constant3/1 -> Product3/1, Product2/3
  Constant20/1 -> Product/3, Product1/1
  TireRadius/1 -> WhlTrqLmt/1
  Add2/1 -> Divide/1
  Constant9/1 -> Add4/2
  Constant7/1 -> Add4/1
  Constant2/1 -> Product/1
  Constant6/1 -> Add3/2
  Mux1/1 -> TireRadius/1
  Divide/1 -> Mux1/1  "Fz_F"
  Add4/1 -> Product1/3
  Add3/1 -> Divide/2
  MaxAcc/1 -> Product1/4, Product3/4  "Ax"
  Constant4/1 -> Product/2, Product1/2
  Constant5/1 -> Add3/1
  Product/1 -> Add2/1
  Product1/1 -> Add2/2

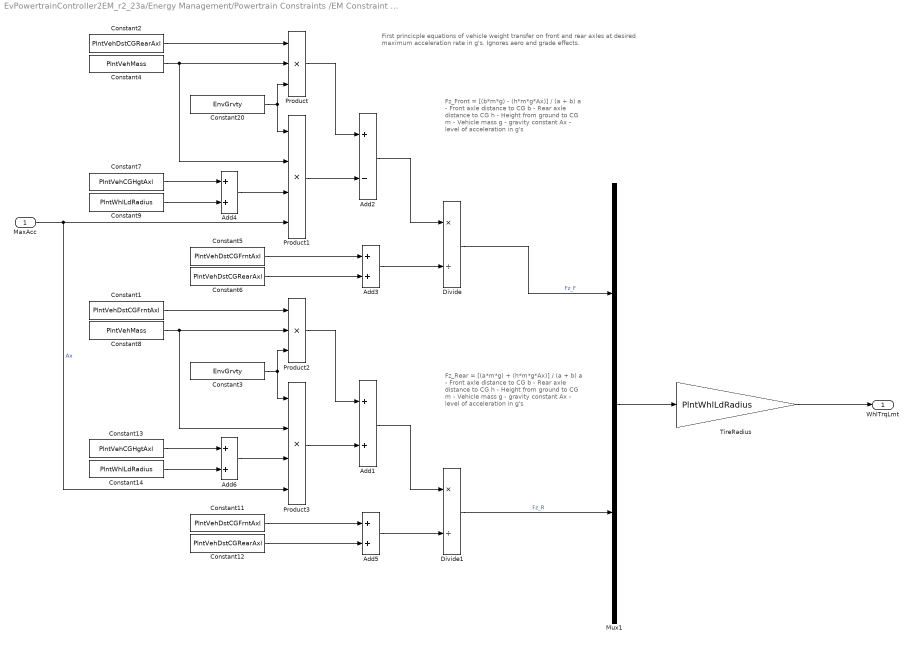
== system EvPowertrainController2EM_r2_23a/Energy Management/Powertrain Constraints /EM Constraint Rear/Wheel Torque Saturation for Max g Rates/Wheel Torque Limit at Max g Rates/Wheel Torque at Max Deceleration Rate ==
  note: First princicple equations of vehicle weight transfer on front
      | and rear axles at desired maximum acceleration rate in g's.
      | Ignores aero and grade effects.
  note: Fz_Front = [(b*m*g) - (h*m*g*Ax)] / (a + b)
      |
      | a - Front axle distance to CG
      | b - Rear axle distance to CG
      | h - Height from ground to CG
      | m - Vehicle mass
      | g - gravity constant
      | Ax - level of acceleration in g's
  note: Fz_Rear = [(a*m*g) + (h*m*g*Ax)] / (a + b)
      |
      | a - Front axle distance to CG
      | b - Rear axle distance to CG
      | h - Height from ground to CG
      | m - Vehicle mass
      | g - gravity constant
      | Ax - level of acceleration in g's
  MaxAcc : Inport
  Add{1,3..6} (5 alike) : Sum
  Add2 : Sum  Inputs=+-
  Constant1 : Constant  Value=PlntVehDstCGFrntAxl  SampleTime=-1
  Constant11 : Constant  Value=PlntVehDstCGFrntAxl  SampleTime=-1
  Constant12 : Constant  Value=PlntVehDstCGRearAxl  SampleTime=-1
  Constant13 : Constant  Value=PlntVehCGHgtAxl  SampleTime=-1
  Constant14 : Constant  Value=PlntWhlLdRadius  SampleTime=-1
  Constant2 : Constant  Value=PlntVehDstCGRearAxl  SampleTime=-1
  Constant20 : Constant  Value=EnvGrvty  SampleTime=-1
  Constant3 : Constant  Value=EnvGrvty  SampleTime=-1
  Constant4 : Constant  Value=PlntVehMass  SampleTime=-1
  Constant5 : Constant  Value=PlntVehDstCGFrntAxl  SampleTime=-1
  Constant6 : Constant  Value=PlntVehDstCGRearAxl  SampleTime=-1
  Constant7 : Constant  Value=PlntVehCGHgtAxl  SampleTime=-1
  Constant8 : Constant  Value=PlntVehMass  SampleTime=-1
  Constant9 : Constant  Value=PlntWhlLdRadius  SampleTime=-1
  Divide : Product  Inputs=*/
  Divide1 : Product  Inputs=*/
  Mux1 : Mux  Inputs=2
  Product : Product  Inputs=3
  Product1 : Product  Inputs=4
  Product2 : Product  Inputs=3
  Product3 : Product  Inputs=4
  TireRadius : Gain  Gain=PlntWhlLdRadius
  WhlTrqLmt : Outport  VectorParamsAs1DForOutWhenUnconnected=off
  wires:
  Product1/1 -> Add2/2
  Product/1 -> Add2/1
  Constant5/1 -> Add3/1
  Constant4/1 -> Product1/2, Product/2
  MaxAcc/1 -> Product3/4, Product1/4  "Ax"
  Add3/1 -> Divide/2
  Add4/1 -> Product1/3
  Divide/1 -> Mux1/1  "Fz_F"
  Mux1/1 -> TireRadius/1
  Constant6/1 -> Add3/2
  Constant2/1 -> Product/1
  Constant7/1 -> Add4/1
  Constant9/1 -> Add4/2
  Add2/1 -> Divide/1
  TireRadius/1 -> WhlTrqLmt/1
  Constant20/1 -> Product1/1, Product/3
  Constant3/1 -> Product2/3, Product3/1
  Add1/1 -> Divide1/1
  Constant14/1 -> Add6/2
  Constant13/1 -> Add6/1
  Constant1/1 -> Product2/1
  Constant12/1 -> Add5/2
  Add6/1 -> Product3/3
  Add5/1 -> Divide1/2
  Constant8/1 -> Product2/2, Product3/2
  Constant11/1 -> Add5/1
  Product2/1 -> Add1/1
  Product3/1 -> Add1/2
  Divide1/1 -> Mux1/2  "Fz_R"

== system EvPowertrainController2EM_r2_23a/Energy Management/Powertrain Constraints /Wheel Torque Vector Logic/Regen/Wheel Torque Max Based on Power Limits/EMTrq2WhlTrq ==
  EMTrqCmd : Inport
  EMSpd : Inport  Port=2
  2EM or 3EM Dual Rear : Subsystem  VariantControl=2EM or 3EM Dual Rear
  3EM Dual Front or 4EM : Subsystem  VariantControl=3EM Dual Front or 4EM
  WhlMotTrq : Outport

== system EvPowertrainController2EM_r2_23a/Energy Management/Powertrain Constraints /Wheel Torque Vector Logic/Regen/Wheel Torque Max Based on Power Limits/Power Management ==
  note: Power Management algorithm:
      | - Estimate Elec power based on mech power using efficiency map
      | - Check if Elec power is within battery power limits
      | - If power within limit , use motor torque command
      | - If power limit exceeded, use limited motor torque
      | - For low Mot Spd, MotPwrReq will be a small number.  Pass through torque command until Mot Spd > 2.
  BattPwrDischrgLmt : Inport
  BattPwrChrgLmt : Inport  Port=2
  EMSpd : Inport  Port=3
  EMTrqCmd : Inport  Port=4
  SOC : Inport  Port=5
  Abs : Abs  SaturateOnIntegerOverflow=off
  Check Within Limits : Subsystem
  Compare To Constant : simulink/Logic and Bit Operations/Compare To Constant  relop=<  const=2  OutDataTypeStr=boolean
  ElecToMechPwr : Product  Inputs=*/
  Mech to Elec Power Estimate : Subsystem
  MechPwrToTrq : Product  Inputs=*/
  Switch : Switch  Criteria=u2 > Threshold  SaturateOnIntegerOverflow=off  InputSameDT=off
  Switch1 : Switch  Criteria=u2 > Threshold  SaturateOnIntegerOverflow=off  InputSameDT=off
  Torque Limit : Subsystem
  div0protect - poly : autolibutils/div0protect - poly  thresh=2  ZeroCross1=off  aMode=6
  EMTrqCmdFinal : Outport  VectorParamsAs1DForOutWhenUnconnected=off
  wires:
  SOC/1 -> Torque Limit/3(SOC)
  Compare To Constant/1 -> Switch1/2
  Abs/1 -> Compare To Constant/1
  Switch1/1 -> Torque Limit/1(EMTrq)
  Check Within Limits/1(InLimit) -> Switch/2
  Switch/1 -> Switch1/3
  Check Within Limits/2(y) -> ElecToMechPwr/1
  BattPwrChrgLmt/1 -> Check Within Limits/3(lo)
  Mech to Elec Power Estimate/1(EMPwrElecReq) -> Check Within Limits/2(u)
  BattPwrDischrgLmt/1 -> Check Within Limits/1(up)
  Torque Limit/1(EMTrqCmd) -> EMTrqCmdFinal/1
  MechPwrToTrq/1 -> Switch/3
  ElecToMechPwr/1 -> MechPwrToTrq/1
  Mech to Elec Power Estimate/2(Eff2k) -> ElecToMechPwr/2
  div0protect - poly/1 -> MechPwrToTrq/2
  EMTrqCmd/1 -> Mech to Elec Power Estimate/1(EMTrqCmd), Switch1/1, Switch/1
  EMSpd/1 -> Mech to Elec Power Estimate/2(EMSpd), div0protect - poly/1, Torque Limit/2(EMSpd), Abs/1

== system EvPowertrainController2EM_r2_23a/Energy Management/Powertrain Constraints /Wheel Torque Vector Logic/Regen/Wheel Torque Max Based on Power Limits/WhlTrq2EMTrq ==
  EMSpd : Inport
  WhlTrqCmd : Inport  Port=2
  2EM or 3EM Dual Rear : Subsystem  VariantControl=2EM or 3EMDualFront
  3EM Dual Front or 4EM : Subsystem  VariantControl=3EM Dual Front or 4EM
  EMTrq : Outport

== system EvPowertrainController2EM_r2_23a/Energy Management/Powertrain Constraints /Wheel Torque Vector Logic/Traction/Wheel Torque Max Based on Power Limits/EMTrq2WhlTrq ==
  EMTrqCmd : Inport
  EMSpd : Inport  Port=2
  2EM or 3EM Dual Front : Subsystem  VariantControl=2EM or 3EM Dual Front
  3EM Dual Rear or 4EM : Subsystem  VariantControl=3EM Dual Rear or 4EM
  WhlMotTrq : Outport

== system EvPowertrainController2EM_r2_23a/Energy Management/Powertrain Constraints /Wheel Torque Vector Logic/Traction/Wheel Torque Max Based on Power Limits/Power Management ==
  note: Power Management algorithm:
      | - Estimate Elec power based on mech power using efficiency map
      | - Check if Elec power is within battery power limits
      | - If power within limit , use motor torque command
      | - If power limit exceeded, use limited motor torque
      | - For low Mot Spd, MotPwrReq will be a small number.  Pass through torque command until Mot Spd > 2.
  BattPwrDischrgLmt : Inport
  BattPwrChrgLmt : Inport  Port=2
  EMSpd : Inport  Port=3
  EMTrqCmd : Inport  Port=4
  SOC : Inport  Port=5
  Abs : Abs  SaturateOnIntegerOverflow=off
  Check Within Limits : Subsystem
  Compare To Constant : simulink/Logic and Bit Operations/Compare To Constant  relop=<  const=2  OutDataTypeStr=boolean
  ElecToMechPwr : Product  Inputs=*/
  Mech to Elec Power Estimate : Subsystem
  MechPwrToTrq : Product  Inputs=*/
  Switch : Switch  Criteria=u2 > Threshold  SaturateOnIntegerOverflow=off  InputSameDT=off
  Switch1 : Switch  Criteria=u2 > Threshold  SaturateOnIntegerOverflow=off  InputSameDT=off
  Torque Limit : Subsystem
  div0protect - poly : autolibutils/div0protect - poly  thresh=2  ZeroCross1=off  aMode=6
  EMTrqCmdFinal : Outport  VectorParamsAs1DForOutWhenUnconnected=off
  wires:
  EMSpd/1 -> Abs/1, Torque Limit/2(EMSpd), div0protect - poly/1, Mech to Elec Power Estimate/2(EMSpd)
  EMTrqCmd/1 -> Switch/1, Switch1/1, Mech to Elec Power Estimate/1(EMTrqCmd)
  div0protect - poly/1 -> MechPwrToTrq/2
  Mech to Elec Power Estimate/2(Eff2k) -> ElecToMechPwr/2
  ElecToMechPwr/1 -> MechPwrToTrq/1
  MechPwrToTrq/1 -> Switch/3
  Torque Limit/1(EMTrqCmd) -> EMTrqCmdFinal/1
  BattPwrDischrgLmt/1 -> Check Within Limits/1(up)
  Mech to Elec Power Estimate/1(EMPwrElecReq) -> Check Within Limits/2(u)
  BattPwrChrgLmt/1 -> Check Within Limits/3(lo)
  Check Within Limits/2(y) -> ElecToMechPwr/1
  Switch/1 -> Switch1/3
  Check Within Limits/1(InLimit) -> Switch/2
  Switch1/1 -> Torque Limit/1(EMTrq)
  Abs/1 -> Compare To Constant/1
  Compare To Constant/1 -> Switch1/2
  SOC/1 -> Torque Limit/3(SOC)

== system EvPowertrainController2EM_r2_23a/Energy Management/Powertrain Constraints /Wheel Torque Vector Logic/Traction/Wheel Torque Max Based on Power Limits/WhlTrq2EMTrq ==
  EMSpd : Inport
  WhlTrqCmd : Inport  Port=2
  2EM or 3EM Dual Front : Subsystem  VariantControl=2EM or 3EM Dual Front
  3EM Dual Rear or 4EM : Subsystem  VariantControl=3EM Dual Rear or 4EM
  EMTrq : Outport

== system EvPowertrainController2EM_r2_23a/Energy Management/Powertrain Constraints /EM Constraint Front/Tabular Power Loss Data/2EM or 3EM Dual Rear/WhlTrq2EMTrq/Diff Eta ==
  note: Pwr >= 0, v = 1
      | Pwr < 0, v= -1
  SpdIn : Inport
  TrqIn : Inport  Port=2
  Constant : Constant  Value=PlntDiffrntl2Eff
  Constant1 : Constant  SampleTime=-1
  Constant2 : Constant  Value=-1  SampleTime=-1
  Math Function1 : Math  Operator=pow  SignedPower=on  OutputSignalType=real
  Product1 : Product
  Switch2 : Switch  SaturateOnIntegerOverflow=off  InputSameDT=off
  eta : Outport  VectorParamsAs1DForOutWhenUnconnected=off
  wires:
  SpdIn/1 -> Product1/2
  Constant/1 -> Math Function1/1
  Constant2/1 -> Switch2/3
  Constant1/1 -> Switch2/1
  Product1/1 -> Switch2/2
  Switch2/1 -> Math Function1/2
  Math Function1/1 -> eta/1
  TrqIn/1 -> Product1/1

== system EvPowertrainController2EM_r2_23a/Energy Management/Powertrain Constraints /EM Constraint Front/Tabular Power Loss Data/3EM Dual Front or 4EM/WhlTrq2EMTrq/Gear Eta ==
  note: Pwr >= 0, v = 1
      | Pwr < 0, v= -1
  SpdIn : Inport
  TrqIn : Inport  Port=2
  Constant : Constant  Value=PlntEMWhlGearEffRL
  Constant1 : Constant  SampleTime=-1
  Constant2 : Constant  Value=-1  SampleTime=-1
  Math Function1 : Math  Operator=pow  SignedPower=on  OutputSignalType=real
  Product1 : Product
  Switch2 : Switch  SaturateOnIntegerOverflow=off  InputSameDT=off
  eta : Outport  VectorParamsAs1DForOutWhenUnconnected=off
  wires:
  TrqIn/1 -> Product1/1
  Math Function1/1 -> eta/1
  Switch2/1 -> Math Function1/2
  Product1/1 -> Switch2/2
  Constant1/1 -> Switch2/1
  Constant2/1 -> Switch2/3
  Constant/1 -> Math Function1/1
  SpdIn/1 -> Product1/2

== system EvPowertrainController2EM_r2_23a/Energy Management/Powertrain Constraints /EM Constraint Rear/Tabular Power Loss Data/2EM/WhlTrq2EMTrq/Diff Eta ==
  note: Pwr >= 0, v = 1
      | Pwr < 0, v= -1
  SpdIn : Inport
  TrqIn : Inport  Port=2
  Constant : Constant  Value=PlntDiffrntl2Eff
  Constant1 : Constant  SampleTime=-1
  Constant2 : Constant  Value=-1  SampleTime=-1
  Math Function1 : Math  Operator=pow  SignedPower=on  OutputSignalType=real
  Product1 : Product
  Switch2 : Switch  SaturateOnIntegerOverflow=off  InputSameDT=off
  eta : Outport  VectorParamsAs1DForOutWhenUnconnected=off
  wires:
  SpdIn/1 -> Product1/2
  Constant/1 -> Math Function1/1
  Constant2/1 -> Switch2/3
  Constant1/1 -> Switch2/1
  Product1/1 -> Switch2/2
  Switch2/1 -> Math Function1/2
  Math Function1/1 -> eta/1
  TrqIn/1 -> Product1/1

== system EvPowertrainController2EM_r2_23a/Energy Management/Powertrain Constraints /EM Constraint Rear/Tabular Power Loss Data/3EM Dual Front/WhlTrq2EMTrq/Diff Eta ==
  note: Pwr >= 0, v = 1
      | Pwr < 0, v= -1
  SpdIn : Inport
  TrqIn : Inport  Port=2
  Constant : Constant  Value=PlntDiffrntl2Eff
  Constant1 : Constant  SampleTime=-1
  Constant2 : Constant  Value=-1  SampleTime=-1
  Math Function1 : Math  Operator=pow  SignedPower=on  OutputSignalType=real
  Product1 : Product
  Switch2 : Switch  SaturateOnIntegerOverflow=off  InputSameDT=off
  eta : Outport  VectorParamsAs1DForOutWhenUnconnected=off
  wires:
  TrqIn/1 -> Product1/1
  Math Function1/1 -> eta/1
  Switch2/1 -> Math Function1/2
  Product1/1 -> Switch2/2
  Constant1/1 -> Switch2/1
  Constant2/1 -> Switch2/3
  Constant/1 -> Math Function1/1
  SpdIn/1 -> Product1/2

== system EvPowertrainController2EM_r2_23a/Energy Management/Powertrain Constraints /EM Constraint Rear/Tabular Power Loss Data/3EM Dual Rear or 4EM/WhlTrq2EMTrq/Gear Eta ==
  note: Pwr >= 0, v = 1
      | Pwr < 0, v= -1
  SpdIn : Inport
  TrqIn : Inport  Port=2
  Constant : Constant  Value=PlntEMWhlGearEffRL
  Constant1 : Constant  SampleTime=-1
  Constant2 : Constant  Value=-1  SampleTime=-1
  Math Function1 : Math  Operator=pow  SignedPower=on  OutputSignalType=real
  Product1 : Product
  Switch2 : Switch  SaturateOnIntegerOverflow=off  InputSameDT=off
  eta : Outport  VectorParamsAs1DForOutWhenUnconnected=off
  wires:
  TrqIn/1 -> Product1/1
  Math Function1/1 -> eta/1
  Switch2/1 -> Math Function1/2
  Product1/1 -> Switch2/2
  Constant1/1 -> Switch2/1
  Constant2/1 -> Switch2/3
  Constant/1 -> Math Function1/1
  SpdIn/1 -> Product1/2

== system EvPowertrainController2EM_r2_23a/Energy Management/Powertrain Constraints /Wheel Torque Vector Logic/Regen/Wheel Torque Max Based on Power Limits/EMTrq2WhlTrq/2EM or 3EM Dual Rear ==
  EMTrqCmd : Inport
  EMSpd : Inport  Port=2
  Diff Eta : Subsystem
  Divide2 : Product  Inputs=**
  Gain3 : Gain  Gain=PlntDiffrntlRatio
  WhlMotTrq : Outport  VectorParamsAs1DForOutWhenUnconnected=off
  wires:
  Gain3/1 -> Divide2/2
  Divide2/1 -> WhlMotTrq/1
  EMSpd/1 -> Diff Eta/1(SpdIn)
  EMTrqCmd/1 -> Diff Eta/2(TrqIn), Gain3/1
  Diff Eta/1(eta) -> Divide2/1

== system EvPowertrainController2EM_r2_23a/Energy Management/Powertrain Constraints /Wheel Torque Vector Logic/Regen/Wheel Torque Max Based on Power Limits/EMTrq2WhlTrq/3EM Dual Front or 4EM ==
  EMTrqCmd : Inport
  EMSpd : Inport  Port=2
  Divide2 : Product  Inputs=**
  Dual EMs : Gain  Gain=2
  Gain3 : Gain  Gain=PlntEMWhlGearRatioFL
  Gear Eta : Subsystem
  WhlMotTrq : Outport  VectorParamsAs1DForOutWhenUnconnected=off
  wires:
  Gain3/1 -> Divide2/2
  Divide2/1 -> WhlMotTrq/1
  EMSpd/1 -> Gear Eta/1(SpdIn)
  EMTrqCmd/1 -> Dual EMs/1
  Gear Eta/1(eta) -> Divide2/1
  Dual EMs/1 -> Gear Eta/2(TrqIn), Gain3/1

== system EvPowertrainController2EM_r2_23a/Energy Management/Powertrain Constraints /Wheel Torque Vector Logic/Regen/Wheel Torque Max Based on Power Limits/Power Management/Check Within Limits ==
  up : Inport
  u : Inport  Port=2
  lo : Inport  Port=3
  Compare To Zero : simulink/Logic and Bit Operations/Compare To Zero  relop=>=  OutDataTypeStr=boolean
  Compare To Zero1 : simulink/Logic and Bit Operations/Compare To Zero  relop=<=  OutDataTypeStr=boolean
  Logical Operator : Logic  AllPortsSameDT=off  OutDataTypeStr=boolean
  Saturation Dynamic1 : simulink/Discontinuities/Saturation Dynamic  OutMin=[]  OutMax=[]  OutDataTypeStr=Inherit: Same as second input  OutDataType=fixdt(1, 16)  OutScaling=2^-10  DoSatur=off
  Subtract : Sum  Inputs=+-
  Subtract1 : Sum  Inputs=-+
  InLimit : Outport  VectorParamsAs1DForOutWhenUnconnected=off
  y : Outport  Port=2  VectorParamsAs1DForOutWhenUnconnected=off
  wires:
  Logical Operator/1 -> InLimit/1
  Compare To Zero1/1 -> Logical Operator/2
  Compare To Zero/1 -> Logical Operator/1
  Subtract1/1 -> Compare To Zero1/1
  Subtract/1 -> Compare To Zero/1
  u/1 -> Saturation Dynamic1/2, Subtract/2, Subtract1/1
  up/1 -> Saturation Dynamic1/1, Subtract/1
  lo/1 -> Saturation Dynamic1/3, Subtract1/2
  Saturation Dynamic1/1 -> y/1
